simulink model "L7task1"  (R2020a)
settings: Solver=VariableStepAuto  StartTime=0.0  StopTime=10.0  RelTol=1e-3
undefined symbols (not defined in the file): b, J, K, L, R
settings Model: Creator=bztig  LastModifiedBy=bztig

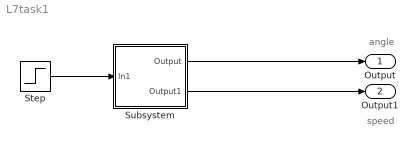
== system L7task1 ==
  note: speed
  note: angle
  Step : Step  After=5  SampleTime=0
  Subsystem : Subsystem
  Output : Outport
  Output1 : Outport  Port=2
  wires:
  Subsystem/1(Output) -> Output/1
  Step/1 -> Subsystem/1(In1)
  Subsystem/2(Output1) -> Output1/1

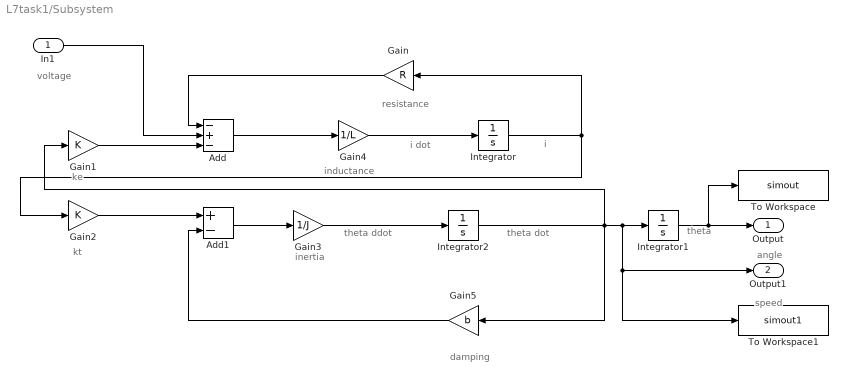
== system L7task1/Subsystem ==
  note: angle
  note: theta
  note: speed
  note: theta dot
  note: theta ddot
  note: damping
  note: resistance
  note: i
  note: i dot
  note: inertia
  note: inductance
  note: kt
  note: ke
  note: voltage
  In1 : Inport
  Add : Sum  Inputs=-+-
  Add1 : Sum  Inputs=+-
  Gain : Gain  Gain=R
  Gain1 : Gain  Gain=K
  Gain2 : Gain  Gain=K
  Gain3 : Gain  Gain=1/J
  Gain4 : Gain  Gain=1/L
  Gain5 : Gain  Gain=b
  Integrator : Integrator
  Integrator1 : Integrator
  Integrator2 : Integrator
  To Workspace : ToWorkspace  VariableName=simout  SampleTime=-1
  To Workspace1 : ToWorkspace  VariableName=simout1  SampleTime=-1
  Output : Outport
  Output1 : Outport  Port=2
  wires:
  Gain5/1 -> Add1/2
  Gain1/1 -> Add/3
  Integrator/1 -> Gain2/1, Gain/1
  Gain2/1 -> Add1/1
  Gain4/1 -> Integrator/1
  Add1/1 -> Gain3/1
  Add/1 -> Gain4/1
  Gain3/1 -> Integrator2/1
  In1/1 -> Add/2
  Integrator2/1 -> Output1/1, To Workspace1/1, Integrator1/1, Gain5/1, Gain1/1
  Gain/1 -> Add/1
  Integrator1/1 -> To Workspace/1, Output/1
